simulink subsystem "Motors"  (R2024b)
settings: Solver=VariableStepAuto  StartTime=0.0  StopTime=10.0  RelTol=1e-3
libraries: stm32l4xxblockslib x2, stm32f4xxblockslib x1
settings Model: Creator=JesseJabezArendse  LastModifiedBy=Nang'alelwa
settings RTWCC: GPUComputeCapability=3.5

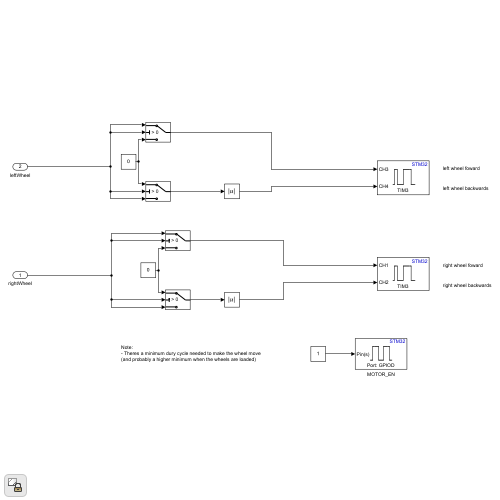
[thumbnail: Simulink's stored preview of the top-level diagram]
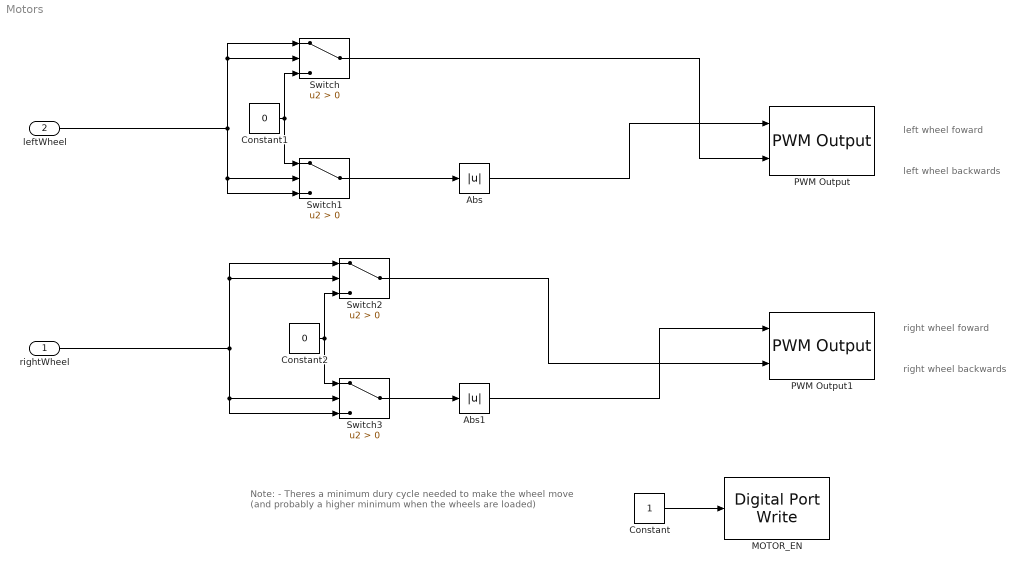
== system Motors ==
  note: Note:
      | - Theres a minimum dury cycle needed to make the wheel move (and probably a higher minimum when the wheels are loaded)
  note: left wheel foward
  note: left wheel backwards
  note: right wheel backwards
  note: right wheel foward
  rightWheel : Inport
  leftWheel : Inport  Port=2
  Abs : Abs  SaturateOnIntegerOverflow=off
  Abs1 : Abs  SaturateOnIntegerOverflow=off
  Constant : Constant
  Constant1 : Constant  Value=0
  Constant2 : Constant  Value=0
  MOTOR_EN : stm32f4xxblockslib/Digital Port Write  PortName=GPIOD  PinNumber=7  ReadOperation=off  IOAsArray=on  EnableSimPort=off  hoistedMaskSrc=ECSoC/ECSimCodegen/Digital Port Write
      settings: LibrarySourceBlock=stm32l4xxblockslib/Digital Port Write
  PWM Output : stm32l4xxblockslib/PWM Output  TimerModule=TIM3  DutycycleUnits=Percentage  EnableChannel1=off  EnableChannel2=off  EnableChannel3=on  EnableChannel4=on  EnableChannel5=off  EnableChannel6=off  EnableCounterInput=off  EnableMainOutputInput=off  EnableFrequencyInput=off  SetRCAfterCE=off  OutputDirection=off  OutputMainOutputEnableStatus=off  SampleTime=0.1  EnableSimPort=off  EnableUpdateEvent=off  EnableCaptureCompare1Event=off  EnableCaptureCompare2Event=off  EnableCaptureCompare3Event=off  EnableCaptureCompare4Event=off  EnableTriggerEvent=off  EnableBreakEvent=off  EnableBreakEvent2=off  ProcessorFamily=STM32L4  hoistedMaskSrc=ECSoC/ECSimCodegen/PWM Output
  PWM Output1 : stm32l4xxblockslib/PWM Output  TimerModule=TIM3  DutycycleUnits=Percentage  EnableChannel1=on  EnableChannel2=on  EnableChannel3=off  EnableChannel4=off  EnableChannel5=off  EnableChannel6=off  EnableCounterInput=off  EnableMainOutputInput=off  EnableFrequencyInput=off  SetRCAfterCE=off  OutputDirection=off  OutputMainOutputEnableStatus=off  SampleTime=0.1  EnableSimPort=off  EnableUpdateEvent=off  EnableCaptureCompare1Event=off  EnableCaptureCompare2Event=off  EnableCaptureCompare3Event=off  EnableCaptureCompare4Event=off  EnableTriggerEvent=off  EnableBreakEvent=off  EnableBreakEvent2=off  ProcessorFamily=STM32L4  hoistedMaskSrc=ECSoC/ECSimCodegen/PWM Output
  Switch{,1..3} (4 alike) : Switch  Criteria=u2 > Threshold  SaturateOnIntegerOverflow=off  InputSameDT=off
  wires:
  Constant/1 -> MOTOR_EN/1
  leftWheel/1 -> Switch1/2, Switch1/3, Switch/2, Switch/1
  Switch/1 -> PWM Output/2
  Switch1/1 -> Abs/1
  Constant1/1 -> Switch1/1, Switch/3
  Constant2/1 -> Switch3/1, Switch2/3
  rightWheel/1 -> Switch2/1, Switch2/2, Switch3/3, Switch3/2
  Switch2/1 -> PWM Output1/2
  Switch3/1 -> Abs1/1
  Abs/1 -> PWM Output/1
  Abs1/1 -> PWM Output1/1
